simulink model "CM475A_TSG31CfgAndUse"  (R2013b)
settings: Solver=FixedStepDiscrete  SolverMode=SingleTasking  StartTime=0.0  StopTime=0.01  FixedStep=0.00005  RelTol=1e-3
values from neighbouring files (symbols this model uses):
  ELECGLBPRM_MOTCTRLINTRPTTRIGCFGB_CNT_U08 = DataDict.Constant    [CM475A_TSG31CfgAndUse_DataDict.m]
  ELECGLBPRM_MOTCTRLINTRPTTRIGSRC_CNT_U08 = DataDict.ConfigParam    [CM475A_TSG31CfgAndUse_DataDict.m]
  ELECGLBPRM_PWMPERDMIN_NANOSEC_U32 = DataDict.ConfigParam    [CM475A_TSG31CfgAndUse_DataDict.m]
  TSG31CfgAndUseAdcStrtOfCnvn2Offs = DataDict.Calibration    [CM475A_TSG31CfgAndUse_DataDict.m]
  TSG31CfgAndUseAdcStrtOfCnvnMotCtrlPeakOffs = DataDict.Calibration    [CM475A_TSG31CfgAndUse_DataDict.m]
  TSG31CfgAndUseAdcStrtOfCnvnMotCtrlVlyOffs = DataDict.Calibration    [CM475A_TSG31CfgAndUse_DataDict.m]
  TSG31CfgAndUseMtrAg0SPIStart = DataDict.Calibration    [CM475A_TSG31CfgAndUse_DataDict.m]
  TSG31CfgAndUsePwmDbnd = DataDict.Calibration    [CM475A_TSG31CfgAndUse_DataDict.m]
  TSG31UPD_NANOSEC_U32 = DataDict.Constant    [CM475A_TSG31CfgAndUse_DataDict.m]
undefined symbols (not defined in the file or in its folder): sigbuilder_block, SysSt1
libraries: simulink x11, CM475A_TSG31CfgAndUse_ModelLibrary_Rev001 x11
(part 5 of 5)

== system CM475A_TSG31CfgAndUse/TSG31CfgAndUse/TSG31CfgAndUsePer2/Transition from Enable/Map FET Ctrl Signals to GPIO and Set Low/Set GPIO Level/IoHwAb_SetGpioPhaCUpprCmd/CopyRight2 ==

== matlab function CM475A_TSG31CfgAndUse/TSG31CfgAndUse/TSG31CfgAndUsePer1/Truth Table ==
  data: MotCurrEolCalSt input uint8; PwmPeriod output uint32; PwmPerd input uint32; PhaOnTiA input uint32; PhaOnTiB input uint32; PhaOnTiC input uint32; PhaseAOnTime output uint32; PhaseBOnTime output uint32; PhaseCOnTime output uint32; CurrMeasEolOffsHiCmuOffs constant uint32; CurrMeasEolFixdPwmPerd constant uint32; CurrMeasEolOffsLoCmuOffs constant double
function [PwmPeriod, PhaseAOnTime, PhaseBOnTime, PhaseCOnTime] = fcn(MotCurrEolCalSt, PwmPerd, PhaOnTiA, PhaOnTiB, PhaOnTiC)

aVarTruthTableCondition_1 = false;
aVarTruthTableCondition_2 = false;
aVarTruthTableCondition_3 = false;
aVarTruthTableCondition_4 = false;


% Normal Operation
% MCECS_OFFSCMDSTRT (0)

aVarTruthTableCondition_1 = logical(MotCurrEolCalSt == 0);

% MCECS_OFFSCMDHI   (1)

aVarTruthTableCondition_2 = logical(MotCurrEolCalSt == 1);

% MCECS_OFFSCMDLO   (2)

aVarTruthTableCondition_3 = logical(MotCurrEolCalSt == 2);

% MCECS_OFFSCMDZERO (3)

aVarTruthTableCondition_4 = logical(MotCurrEolCalSt == 3);

if (aVarTruthTableCondition_2)
    aFcnTruthTableAction_1();
elseif (aVarTruthTableCondition_3)
    aFcnTruthTableAction_2();
elseif (aVarTruthTableCondition_4)
    aFcnTruthTableAction_3();
elseif (aVarTruthTableCondition_1)
    aFcnTruthTableAction_4();
else % Default
    aFcnTruthTableAction_4();
end

function aFcnTruthTableAction_1()

% MCECS_OFFSCMDHI   (1)

PwmPeriod = uint32(CurrMeasEolFixdPwmPerd);
PhaseAOnTime = uint32(CurrMeasEolOffsHiCmuOffs);
PhaseBOnTime = uint32(CurrMeasEolOffsHiCmuOffs);
PhaseCOnTime = uint32(CurrMeasEolOffsHiCmuOffs);

function aFcnTruthTableAction_2()

% MCECS_OFFSCMDLO   (2)

PwmPeriod = uint32(CurrMeasEolFixdPwmPerd);
PhaseAOnTime = uint32(CurrMeasEolOffsLoCmuOffs);
PhaseBOnTime = uint32(CurrMeasEolOffsLoCmuOffs);
PhaseCOnTime = uint32(CurrMeasEolOffsLoCmuOffs);

function aFcnTruthTableAction_3()

% MCECS_OFFSCMDZERO (3)

PwmPeriod = uint32(CurrMeasEolFixdPwmPerd);
PhaseAOnTime = uint32(0);
PhaseBOnTime = uint32(0);
PhaseCOnTime = uint32(0);

function aFcnTruthTableAction_4()

% Default

PwmPeriod = uint32(PwmPerd);
PhaseAOnTime = uint32(PhaOnTiA);
PhaseBOnTime = uint32(PhaOnTiB);
PhaseCOnTime = uint32(PhaOnTiC);

== matlab function CM475A_TSG31CfgAndUse/TSG31CfgAndUse/TSG31CfgAndUsePer2/Truth Table ==
  data: SysStateEnable input boolean; Out1 output; PrevSysStateEnable input boolean
function Out1 = fcn(SysStateEnable, PrevSysStateEnable)

aVarTruthTableCondition_1 = false;
aVarTruthTableCondition_2 = false;


% SysState = Enable

aVarTruthTableCondition_1 = logical(SysStateEnable == 1);

% PrevSysState = Enable

aVarTruthTableCondition_2 = logical(PrevSysStateEnable == 1);

if (aVarTruthTableCondition_1 && aVarTruthTableCondition_2)
    aFcnTruthTableAction_1();
elseif (~aVarTruthTableCondition_1 && aVarTruthTableCondition_2)
    aFcnTruthTableAction_2();
elseif (aVarTruthTableCondition_1 && ~aVarTruthTableCondition_2)
    aFcnTruthTableAction_3();
else % Default
    aFcnTruthTableAction_4();
end

function aFcnTruthTableAction_1()

% No Transition
% SysState = Enable

Out1 = 1;

function aFcnTruthTableAction_2()

% Transition from Enable

Out1 = 2;

function aFcnTruthTableAction_3()

% Transition to Enable

Out1 = 3;

function aFcnTruthTableAction_4()

% No Transition
% SysState != Enable

Out1 = 4;
